simulink model "Exp5_AtoD_Soham_19EE10075"  (R2020b)
settings: Solver=VariableStepAuto  StartTime=0.0  StopTime=10.0  RelTol=1e-3
libraries: powerlib x40, powerlib_meascontrol x10
settings Model: Creator=User  LastModifiedBy=User

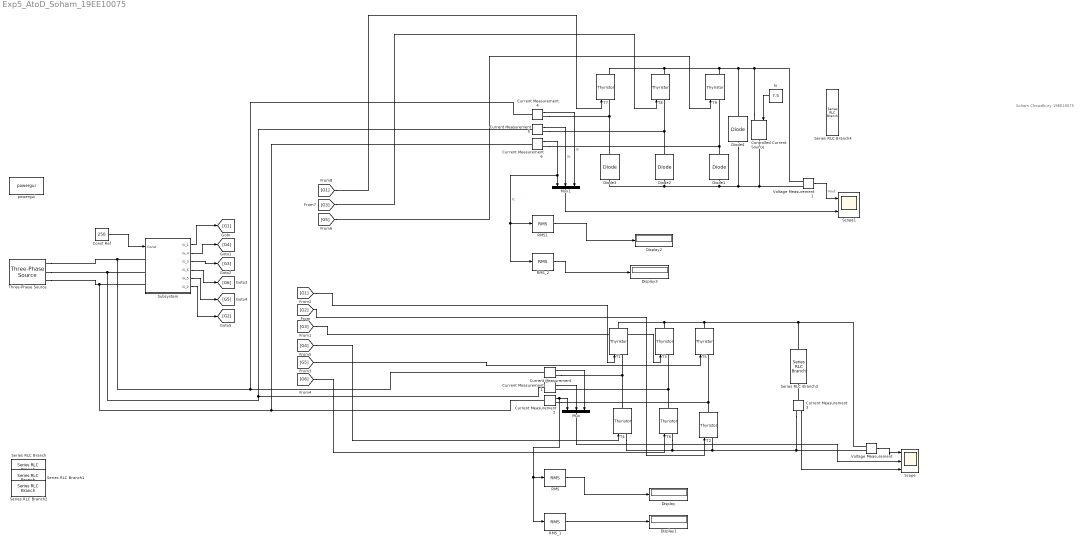
== system Exp5_AtoD_Soham_19EE10075 ==
  note: Soham Chowdhury
      | 19EE10075
  Const Ref : Constant  Value=250
  Controlled Current Source : powerlib/Electrical Sources/Controlled Current Source  Initialize=on  Source_Type=DC  Amplitude=7.5  Phase=0  Frequency=0  Measurements=None
  Current Measurement{,1..6} (7 alike) : powerlib/Measurements/Current Measurement  PhasorSimulation=off  OutputType=Complex  PSBequivalent=0
  Diode{1..4} (4 alike) : powerlib/Power Electronics/Diode  Ron=1e-3  Lon=0  Vf=0  IC=0  UseSnubber=0  Rs=1e12  Cs=inf  Measurements=off
  Display{,1..3} (4 alike) : Display
  Io : Constant  Value=7.5
  Mux : Mux  Inputs=3
  Mux1 : Mux  Inputs=3
  RMS : powerlib_meascontrol/Measurements/RMS  TrueRMS=on  Freq=50  RMSInit=0  Ts=0
  RMS1 : powerlib_meascontrol/Measurements/RMS  TrueRMS=on  Freq=50  RMSInit=0  Ts=0
  RMS_1 : powerlib_meascontrol/Measurements/RMS  TrueRMS=off  Freq=50  RMSInit=0  Ts=0
  RMS_2 : powerlib_meascontrol/Measurements/RMS  TrueRMS=off  Freq=50  RMSInit=0  Ts=0
  Scope : Scope  NumInputPorts=3
  Scope1 : Scope  NumInputPorts=2
  Series RLC Branch : powerlib/Elements/Series RLC Branch  LConnTagsString=__new0  RConnTagsString=__new0  BranchType=L  Resistance=1  Inductance=5e-3  SetiL0=off  InitialCurrent=0  Capacitance=1e-6  Setx0=off  InitialVoltage=0  Measurements=None
  Series RLC Branch1 : powerlib/Elements/Series RLC Branch  LConnTagsString=__new0  RConnTagsString=__new0  BranchType=L  Resistance=1  Inductance=5e-3  SetiL0=off  InitialCurrent=0  Capacitance=1e-6  Setx0=off  InitialVoltage=0  Measurements=None
  Series RLC Branch2 : powerlib/Elements/Series RLC Branch  LConnTagsString=__new0  RConnTagsString=__new0  BranchType=L  Resistance=1  Inductance=5e-3  SetiL0=off  InitialCurrent=0  Capacitance=1e-6  Setx0=off  InitialVoltage=0  Measurements=None
  Series RLC Branch3 : powerlib/Elements/Series RLC Branch  LConnTagsString=__new0  RConnTagsString=__new0  BranchType=RL  Resistance=1  Inductance=60e-3  SetiL0=off  InitialCurrent=0  Capacitance=1e-6  Setx0=off  InitialVoltage=0  Measurements=None
  Series RLC Branch4 : powerlib/Elements/Series RLC Branch  LConnTagsString=__new0  RConnTagsString=__new0  BranchType=RL  Resistance=29.18  Inductance=50e-3  SetiL0=off  InitialCurrent=0  Capacitance=1e-6  Setx0=off  InitialVoltage=0  Measurements=None
  Subsystem : Subsystem
  T{1..6} (6 alike) : powerlib/Power Electronics/Thyristor  Ron=1e-3  Lon=0  Vf=0  IC=0  Rs=1e12  Cs=inf  Measurements=off
  T7 : powerlib/Power Electronics/Thyristor  Ron=1e-3  Lon=0  Vf=0  IC=0  Rs=1e12  Cs=inf  Measurements=on
  T8 : powerlib/Power Electronics/Thyristor  Ron=1e-3  Lon=0  Vf=0  IC=0  Rs=1e12  Cs=inf  Measurements=on
  T9 : powerlib/Power Electronics/Thyristor  Ron=1e-3  Lon=0  Vf=0  IC=0  Rs=1e12  Cs=inf  Measurements=on
  Three-Phase Source : powerlib/Electrical Sources/Three-Phase Source  InternalConnection=Y  VoltagePhases=off  Voltage=220  PhaseAngle=0  Voltage_phases=[25e3 25e3 25e3]/sqrt(3)  PhaseAngles_phases=[0 -120 +120]  Frequency=50  NonIdealSource=on  SpecifyImpedance=off  Resistance=0  Inductance=0  ShortCircuitLevel=100e6  BaseVoltage=220  XRratio=7  BusType=swing  Pref=10e3  Qref=0  Prefabc=[10e3, 10e3, 10e3]  Qrefabc=[0, 0, 0]  Qmin=-inf  Qmax=inf
  Voltage Measurement : powerlib/Measurements/Voltage Measurement  PhasorSimulation=off  OutputType=Complex  PSBequivalent=0
  Voltage Measurement1 : powerlib/Measurements/Voltage Measurement  PhasorSimulation=off  OutputType=Complex  PSBequivalent=0
  powergui : powerlib/powergui  Priority=1  SimulationMode=Continuous  SampleTime=1e-9  frequency=60  Iterations=50  frequencyindice=50  Pbase=100e6  ErrMax=1e-4  UnitsV=kV  UnitsW=MW  buscounter=0  FunctionMessages=off  echomessages=off  EnableUseOfTLC=off  CurrentSourceSwitches=off  DisableSnubberDevices=off  DisableRonSwitches=off  DisableVfSwitches=off  DisplayEquations=off  AutomaticDiscreteSolvers=off  SolverType=Tustin/Backward Euler (TBE)  Interpol=off  ExternalGateDelay=off  methode=off  Ts=100  x0status=blocks  SPID=on  SwTol=0  HookPort=off  NonlinearTolerance=1e-4  nMaxIteration=100  ContinueOnMaxIteration=off  RestoreLinks=warning  ResistiveCurrentMeasurement=off  Frange=[0:2:500]  Ylog=off  Xlog=on  ShowGrid=off  save=off  variable=ZData  structure=0  ZoomFFT=off  StartTime=0.0  cycles=1  DisplayStyle=1  fundamental=60  FreqAxis=off  MaxFrequency=1000  frequencyindicesteady=1  RmsSteady=1  display=off
  wires:
  [G1] -> T7/1
  RMS_2/1 -> Display3/1
  Voltage Measurement1/1 -> Scope1/1  "Vout"
  Current Measurement4/1 -> Mux1/3  "Ia"
  Mux1/1 -> Scope1/2
  Current Measurement6/1 -> RMS1/1, RMS_2/1, Mux1/1  "Ic"
  Io/1 -> Controlled Current Source/1
  [G5] -> T9/1
  [G2] -> T2/1
  [G1] -> T1/1
  Mux/1 -> Scope/2
  Current Measurement1/1 -> Mux/2
  Current Measurement3/1 -> Scope/3
  Current Measurement5/1 -> Mux1/2  "Ib"
  RMS_1/1 -> Display1/1
  RMS/1 -> Display/1
  [G5] -> T5/1
  [G4] -> T4/1
  Current Measurement/1 -> Mux/3
  RMS1/1 -> Display2/1
  Current Measurement2/1 -> Mux/1, RMS_1/1, RMS/1
  Subsystem/6(G_2) -> [G2]
  Subsystem/2(G_4) -> [G4]
  Subsystem/5(G_5) -> [G5]
  Subsystem/1(G_1) -> [G1]
  Const Ref/1 -> Subsystem/1(Const)
  Voltage Measurement/1 -> Scope/1
  Subsystem/3(G_3) -> [G3]
  Subsystem/4(G_6) -> [G6]
  [G6] -> T6/1
  [G3] -> T8/1
  [G3] -> T3/1
  connections:
  Controlled Current Source/LConn1 -- Voltage Measurement1/LConn1 -- Diode4/RConn1 -- T7/RConn1 -- T8/RConn1 -- T9/RConn1
  Diode1/LConn1 -- Voltage Measurement1/LConn2 -- Controlled Current Source/RConn1 -- Diode4/LConn1 -- Diode2/LConn1 -- Diode3/LConn1
  Current Measurement6/RConn1 -- Diode1/RConn1 -- T9/LConn1
  T1/RConn1 -- T3/RConn1 -- T5/RConn1 -- Series RLC Branch3/LConn1 -- Voltage Measurement/LConn1
  T1/LConn1 -- T4/RConn1 -- Current Measurement/RConn1
  Current Measurement1/LConn1 -- Current Measurement5/LConn1 -- Subsystem/LConn2 -- Three-Phase Source/RConn2
  T2/LConn1 -- Voltage Measurement/LConn2 -- Current Measurement3/RConn1 -- T4/LConn1 -- T6/LConn1
  Three-Phase Source/RConn1 -- Current Measurement4/LConn1 -- Current Measurement/LConn1 -- Subsystem/LConn1
  T5/LConn1 -- T2/RConn1 -- Current Measurement2/RConn1
  Three-Phase Source/RConn3 -- Current Measurement6/LConn1 -- Current Measurement2/LConn1 -- Subsystem/LConn3
  Current Measurement5/RConn1 -- T8/LConn1 -- Diode2/RConn1
  Current Measurement4/RConn1 -- T7/LConn1 -- Diode3/RConn1
  T3/LConn1 -- T6/RConn1 -- Current Measurement1/RConn1
  Current Measurement3/LConn1 -- Series RLC Branch3/RConn1

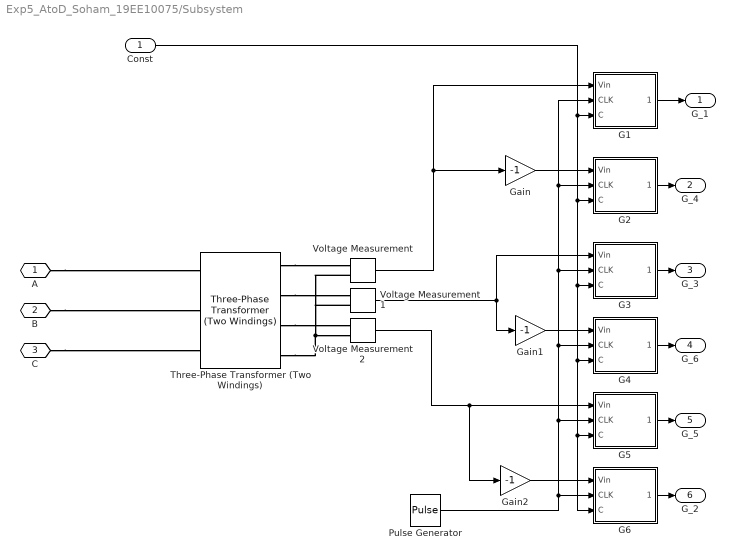
== system Exp5_AtoD_Soham_19EE10075/Subsystem ==
  Const : Inport
  G1 : Subsystem
  G2 : Subsystem
  G3 : Subsystem
  G4 : Subsystem
  G5 : Subsystem
  G6 : Subsystem
  Gain : Gain  Gain=-1
  Gain1 : Gain  Gain=-1
  Gain2 : Gain  Gain=-1
  Pulse Generator : DiscretePulseGenerator  PulseType=Time based  Period=1e-5  PulseWidth=50
  Three-Phase Transformer (Two Windings) : powerlib/Elements/Three-Phase Transformer (Two Windings)  Winding1Connection=Y  Winding2Connection=Yn  CoreType=Three single-phase transformers  SetSaturation=off  Hysteresis=off  DataFile='hysteresis'  SetInitialFlux=off  Measurements=None  UNITS=SI  NominalPower=[100 , 50 ]  Winding1=[220*sqrt(2) 0 0]  Winding2=[5*sqrt(3) 0 0]  Rm=1e6  Lm=1e6  L0=2.866  Saturation=[0 0;0.66653 1910.3;277.72 2419.7]  InitialFluxes=[1273.5 -1273.5 1114.3]  BreakLoop=off  DiscreteSolver=Trapezoidal iterative  DataType=on  TransfoNumber=1
  Voltage Measurement : powerlib/Measurements/Voltage Measurement  PhasorSimulation=off  OutputType=Complex  PSBequivalent=0
  Voltage Measurement1 : powerlib/Measurements/Voltage Measurement  PhasorSimulation=off  OutputType=Complex  PSBequivalent=0
  Voltage Measurement2 : powerlib/Measurements/Voltage Measurement  PhasorSimulation=off  OutputType=Complex  PSBequivalent=0
  A : PMIOPort  Side=Left
  B : PMIOPort  Port=2  Side=Left
  C : PMIOPort  Port=3  Side=Left
  G_1 : Outport
  G_4 : Outport  Port=2
  G_3 : Outport  Port=3
  G_6 : Outport  Port=4
  G_5 : Outport  Port=5
  G_2 : Outport  Port=6
  wires:
  Voltage Measurement/1 -> Gain/1, G1/1(Vin)
  Voltage Measurement2/1 -> G5/1(Vin), Gain2/1
  Const/1 -> G2/3(C), G3/3(C), G4/3(C), G6/3(C), G5/3(C), G1/3(C)
  G2/1(Outport) -> G_4/1
  Pulse Generator/1 -> G6/2(CLK), G5/2(CLK), G4/2(CLK), G3/2(CLK), G2/2(CLK), G1/2(CLK)
  G4/1(Outport) -> G_6/1
  Voltage Measurement1/1 -> G3/1(Vin), Gain1/1
  G6/1(Outport) -> G_2/1
  Gain2/1 -> G6/1(Vin)
  Gain/1 -> G2/1(Vin)
  Gain1/1 -> G4/1(Vin)
  G3/1(Outport) -> G_3/1
  G5/1(Outport) -> G_5/1
  G1/1(Outport) -> G_1/1
  connections:
  Three-Phase Transformer (Two Windings)/RConn1 -- Voltage Measurement/LConn1
  Three-Phase Transformer (Two Windings)/RConn4 -- Voltage Measurement/LConn2 -- Voltage Measurement1/LConn2 -- Voltage Measurement2/LConn2
  Three-Phase Transformer (Two Windings)/RConn2 -- Voltage Measurement1/LConn1
  B/RConn1 -- Three-Phase Transformer (Two Windings)/LConn2
  Three-Phase Transformer (Two Windings)/RConn3 -- Voltage Measurement2/LConn1
  C/RConn1 -- Three-Phase Transformer (Two Windings)/LConn3
  A/RConn1 -- Three-Phase Transformer (Two Windings)/LConn1

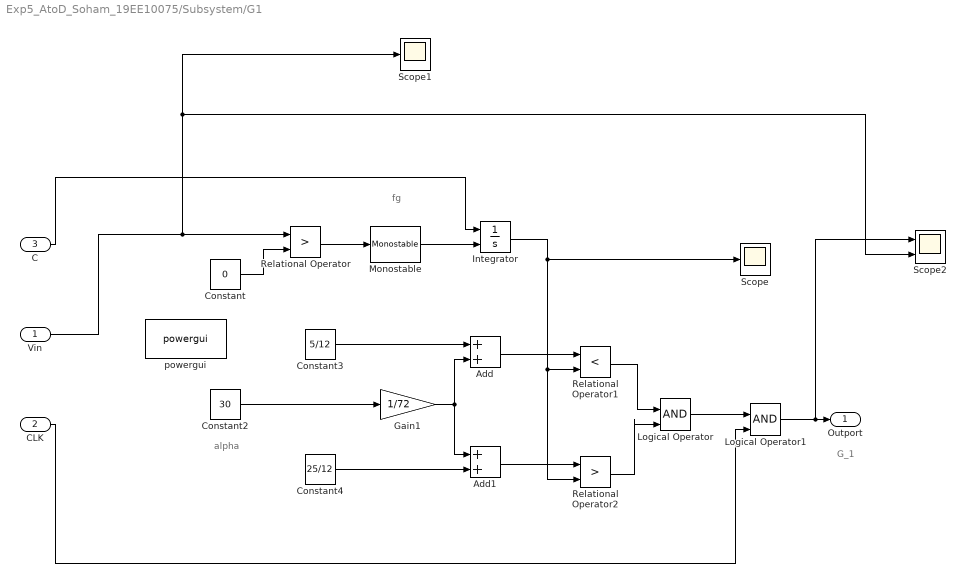
== system Exp5_AtoD_Soham_19EE10075/Subsystem/G1 ==
  note: G_1
  note: alpha
  note: fg
  Vin : Inport
  CLK : Inport  Port=2
  C : Inport  Port=3
  Add : Sum
  Add1 : Sum
  Constant : Constant  Value=0
  Constant2 : Constant  Value=30
  Constant3 : Constant  Value=5/12
  Constant4 : Constant  Value=25/12
  Gain1 : Gain  Gain=1/72
  Integrator : Integrator  ExternalReset=rising
  Logical Operator : Logic  IconShape=distinctive  AllPortsSameDT=off  OutDataTypeStr=boolean
  Logical Operator1 : Logic  IconShape=distinctive  AllPortsSameDT=off  OutDataTypeStr=boolean
  Monostable : powerlib_meascontrol/Logic/Monostable  EdgeDetect=Rising  PulseDuration=1e-05  ic=0  Ts=0
      settings: SourceProductBaseCode=PS
  Relational Operator : RelationalOperator  Operator=>  OutDataTypeStr=boolean  RndMeth=Simplest
  Relational Operator1 : RelationalOperator  Operator=<  OutDataTypeStr=boolean  RndMeth=Simplest
  Relational Operator2 : RelationalOperator  Operator=>  OutDataTypeStr=boolean  RndMeth=Simplest
  Scope : Scope
  Scope1 : Scope
  Scope2 : Scope  NumInputPorts=2
  powergui : powerlib/powergui  Priority=1  SimulationMode=Discrete  SampleTime=1e-9  frequency=60  Iterations=50  frequencyindice=60  Pbase=100e6  ErrMax=1e-4  UnitsV=kV  UnitsW=MW  buscounter=0  FunctionMessages=off  echomessages=off  EnableUseOfTLC=off  CurrentSourceSwitches=off  DisableSnubberDevices=off  DisableRonSwitches=off  DisableVfSwitches=off  DisplayEquations=off  AutomaticDiscreteSolvers=off  SolverType=Tustin/Backward Euler (TBE)  Interpol=off  ExternalGateDelay=off  methode=off  Ts=100  x0status=blocks  SPID=on  SwTol=0  HookPort=off  NonlinearTolerance=1e-4  nMaxIteration=100  ContinueOnMaxIteration=off  RestoreLinks=warning  ResistiveCurrentMeasurement=off  Frange=[0:2:500]  Ylog=off  Xlog=on  ShowGrid=off  save=off  variable=ZData  structure=0  ZoomFFT=off  StartTime=0.0  cycles=1  DisplayStyle=1  fundamental=60  FreqAxis=off  MaxFrequency=1000  frequencyindicesteady=1  RmsSteady=1  display=off
  Outport : Outport
  wires:
  Add1/1 -> Relational Operator2/1
  Integrator/1 -> Relational Operator2/2, Relational Operator1/2, Scope/1
  Relational Operator/1 -> Monostable/1
  Add/1 -> Relational Operator1/1
  Constant/1 -> Relational Operator/2
  Relational Operator2/1 -> Logical Operator/2
  Constant3/1 -> Add/1
  Gain1/1 -> Add1/1, Add/2
  Constant4/1 -> Add1/2
  Logical Operator/1 -> Logical Operator1/1
  Monostable/1 -> Integrator/2
  Relational Operator1/1 -> Logical Operator/1
  Logical Operator1/1 -> Scope2/1, Outport/1
  Vin/1 -> Scope2/2, Scope1/1, Relational Operator/1
  CLK/1 -> Logical Operator1/2
  C/1 -> Integrator/1
  Constant2/1 -> Gain1/1

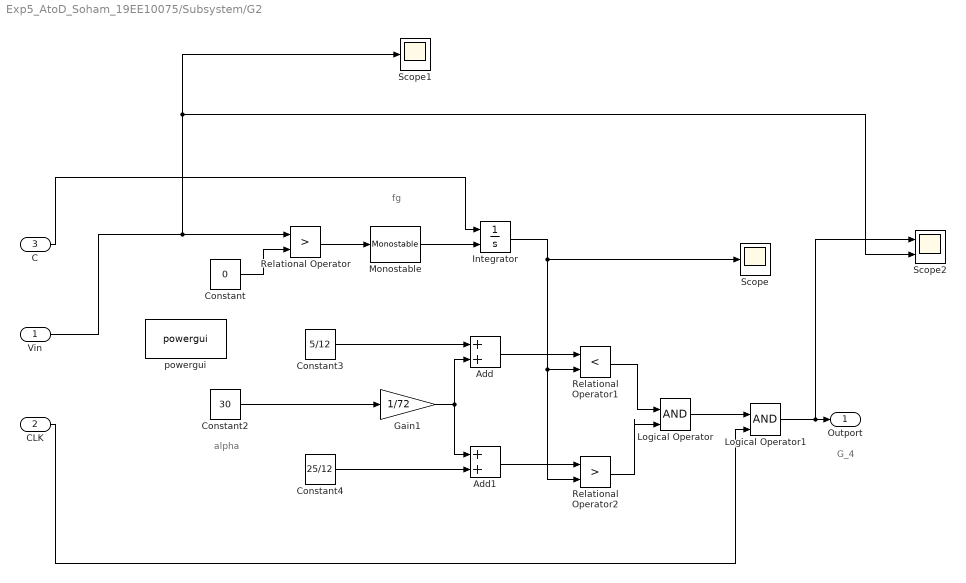
== system Exp5_AtoD_Soham_19EE10075/Subsystem/G2 ==
  note: G_4
  note: alpha
  note: fg
  Vin : Inport
  CLK : Inport  Port=2
  C : Inport  Port=3
  Add : Sum
  Add1 : Sum
  Constant : Constant  Value=0
  Constant2 : Constant  Value=30
  Constant3 : Constant  Value=5/12
  Constant4 : Constant  Value=25/12
  Gain1 : Gain  Gain=1/72
  Integrator : Integrator  ExternalReset=rising
  Logical Operator : Logic  IconShape=distinctive  AllPortsSameDT=off  OutDataTypeStr=boolean
  Logical Operator1 : Logic  IconShape=distinctive  AllPortsSameDT=off  OutDataTypeStr=boolean
  Monostable : powerlib_meascontrol/Logic/Monostable  EdgeDetect=Rising  PulseDuration=1e-05  ic=0  Ts=0
      settings: SourceProductBaseCode=PS
  Relational Operator : RelationalOperator  Operator=>  OutDataTypeStr=boolean  RndMeth=Simplest
  Relational Operator1 : RelationalOperator  Operator=<  OutDataTypeStr=boolean  RndMeth=Simplest
  Relational Operator2 : RelationalOperator  Operator=>  OutDataTypeStr=boolean  RndMeth=Simplest
  Scope : Scope
  Scope1 : Scope
  Scope2 : Scope  NumInputPorts=2
  powergui : powerlib/powergui  Priority=1  SimulationMode=Discrete  SampleTime=1e-9  frequency=60  Iterations=50  frequencyindice=60  Pbase=100e6  ErrMax=1e-4  UnitsV=kV  UnitsW=MW  buscounter=0  FunctionMessages=off  echomessages=off  EnableUseOfTLC=off  CurrentSourceSwitches=off  DisableSnubberDevices=off  DisableRonSwitches=off  DisableVfSwitches=off  DisplayEquations=off  AutomaticDiscreteSolvers=off  SolverType=Tustin/Backward Euler (TBE)  Interpol=off  ExternalGateDelay=off  methode=off  Ts=100  x0status=blocks  SPID=on  SwTol=0  HookPort=off  NonlinearTolerance=1e-4  nMaxIteration=100  ContinueOnMaxIteration=off  RestoreLinks=warning  ResistiveCurrentMeasurement=off  Frange=[0:2:500]  Ylog=off  Xlog=on  ShowGrid=off  save=off  variable=ZData  structure=0  ZoomFFT=off  StartTime=0.0  cycles=1  DisplayStyle=1  fundamental=60  FreqAxis=off  MaxFrequency=1000  frequencyindicesteady=1  RmsSteady=1  display=off
  Outport : Outport
  wires:
  Add1/1 -> Relational Operator2/1
  Integrator/1 -> Relational Operator2/2, Relational Operator1/2, Scope/1
  Relational Operator/1 -> Monostable/1
  Add/1 -> Relational Operator1/1
  Constant/1 -> Relational Operator/2
  Relational Operator2/1 -> Logical Operator/2
  Constant3/1 -> Add/1
  Gain1/1 -> Add1/1, Add/2
  Constant4/1 -> Add1/2
  Logical Operator/1 -> Logical Operator1/1
  Monostable/1 -> Integrator/2
  Relational Operator1/1 -> Logical Operator/1
  Logical Operator1/1 -> Scope2/1, Outport/1
  Vin/1 -> Scope2/2, Scope1/1, Relational Operator/1
  CLK/1 -> Logical Operator1/2
  C/1 -> Integrator/1
  Constant2/1 -> Gain1/1

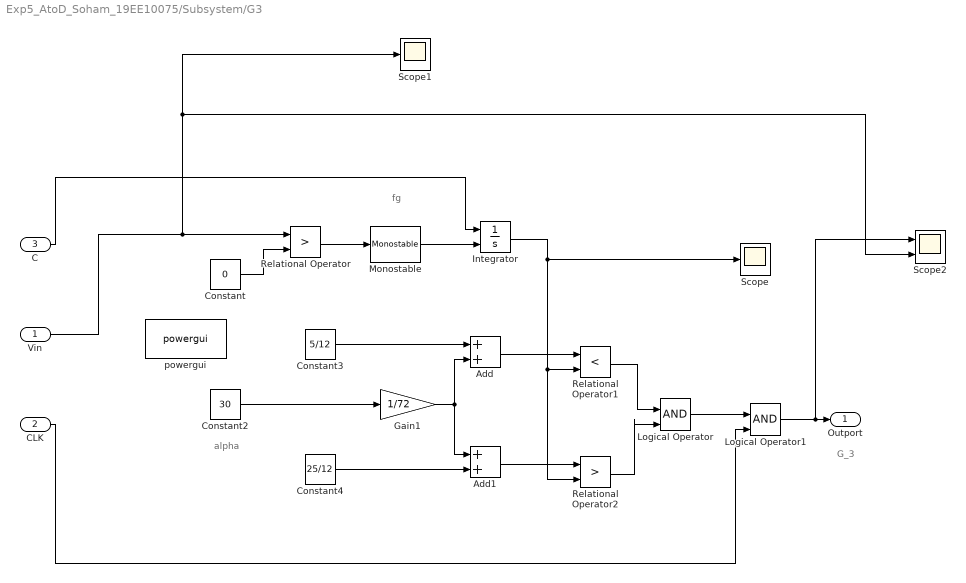
== system Exp5_AtoD_Soham_19EE10075/Subsystem/G3 ==
  note: G_3
  note: alpha
  note: fg
  Vin : Inport
  CLK : Inport  Port=2
  C : Inport  Port=3
  Add : Sum
  Add1 : Sum
  Constant : Constant  Value=0
  Constant2 : Constant  Value=30
  Constant3 : Constant  Value=5/12
  Constant4 : Constant  Value=25/12
  Gain1 : Gain  Gain=1/72
  Integrator : Integrator  ExternalReset=rising
  Logical Operator : Logic  IconShape=distinctive  AllPortsSameDT=off  OutDataTypeStr=boolean
  Logical Operator1 : Logic  IconShape=distinctive  AllPortsSameDT=off  OutDataTypeStr=boolean
  Monostable : powerlib_meascontrol/Logic/Monostable  EdgeDetect=Rising  PulseDuration=1e-05  ic=0  Ts=0
      settings: SourceProductBaseCode=PS
  Relational Operator : RelationalOperator  Operator=>  OutDataTypeStr=boolean  RndMeth=Simplest
  Relational Operator1 : RelationalOperator  Operator=<  OutDataTypeStr=boolean  RndMeth=Simplest
  Relational Operator2 : RelationalOperator  Operator=>  OutDataTypeStr=boolean  RndMeth=Simplest
  Scope : Scope
  Scope1 : Scope
  Scope2 : Scope  NumInputPorts=2
  powergui : powerlib/powergui  Priority=1  SimulationMode=Discrete  SampleTime=1e-9  frequency=60  Iterations=50  frequencyindice=60  Pbase=100e6  ErrMax=1e-4  UnitsV=kV  UnitsW=MW  buscounter=0  FunctionMessages=off  echomessages=off  EnableUseOfTLC=off  CurrentSourceSwitches=off  DisableSnubberDevices=off  DisableRonSwitches=off  DisableVfSwitches=off  DisplayEquations=off  AutomaticDiscreteSolvers=off  SolverType=Tustin/Backward Euler (TBE)  Interpol=off  ExternalGateDelay=off  methode=off  Ts=100  x0status=blocks  SPID=on  SwTol=0  HookPort=off  NonlinearTolerance=1e-4  nMaxIteration=100  ContinueOnMaxIteration=off  RestoreLinks=warning  ResistiveCurrentMeasurement=off  Frange=[0:2:500]  Ylog=off  Xlog=on  ShowGrid=off  save=off  variable=ZData  structure=0  ZoomFFT=off  StartTime=0.0  cycles=1  DisplayStyle=1  fundamental=60  FreqAxis=off  MaxFrequency=1000  frequencyindicesteady=1  RmsSteady=1  display=off
  Outport : Outport
  wires:
  Add1/1 -> Relational Operator2/1
  Integrator/1 -> Relational Operator2/2, Relational Operator1/2, Scope/1
  Relational Operator/1 -> Monostable/1
  Add/1 -> Relational Operator1/1
  Constant/1 -> Relational Operator/2
  Relational Operator2/1 -> Logical Operator/2
  Constant3/1 -> Add/1
  Gain1/1 -> Add1/1, Add/2
  Constant4/1 -> Add1/2
  Logical Operator/1 -> Logical Operator1/1
  Monostable/1 -> Integrator/2
  Relational Operator1/1 -> Logical Operator/1
  Logical Operator1/1 -> Scope2/1, Outport/1
  Vin/1 -> Scope2/2, Scope1/1, Relational Operator/1
  CLK/1 -> Logical Operator1/2
  C/1 -> Integrator/1
  Constant2/1 -> Gain1/1

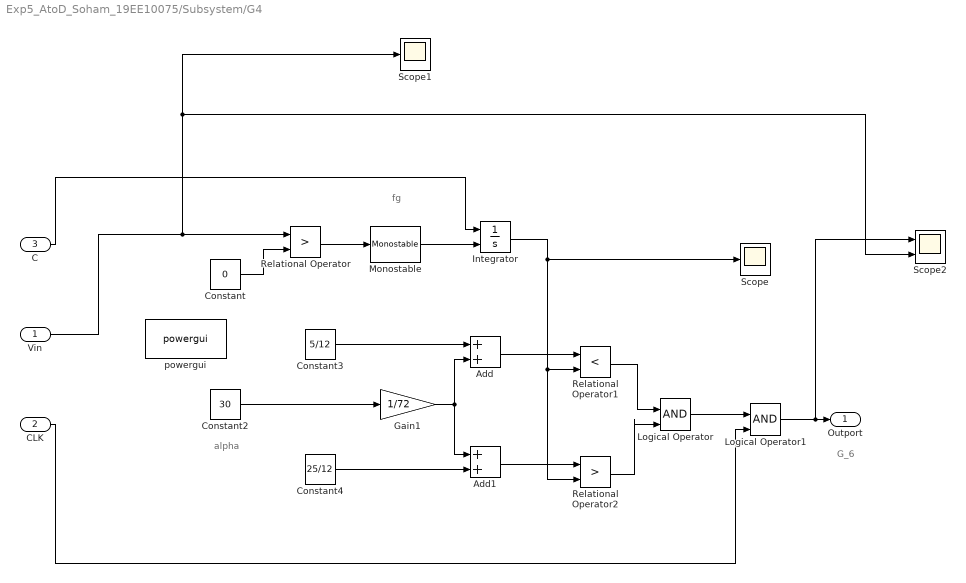
== system Exp5_AtoD_Soham_19EE10075/Subsystem/G4 ==
  note: G_6
  note: alpha
  note: fg
  Vin : Inport
  CLK : Inport  Port=2
  C : Inport  Port=3
  Add : Sum
  Add1 : Sum
  Constant : Constant  Value=0
  Constant2 : Constant  Value=30
  Constant3 : Constant  Value=5/12
  Constant4 : Constant  Value=25/12
  Gain1 : Gain  Gain=1/72
  Integrator : Integrator  ExternalReset=rising
  Logical Operator : Logic  IconShape=distinctive  AllPortsSameDT=off  OutDataTypeStr=boolean
  Logical Operator1 : Logic  IconShape=distinctive  AllPortsSameDT=off  OutDataTypeStr=boolean
  Monostable : powerlib_meascontrol/Logic/Monostable  EdgeDetect=Rising  PulseDuration=1e-05  ic=0  Ts=0
      settings: SourceProductBaseCode=PS
  Relational Operator : RelationalOperator  Operator=>  OutDataTypeStr=boolean  RndMeth=Simplest
  Relational Operator1 : RelationalOperator  Operator=<  OutDataTypeStr=boolean  RndMeth=Simplest
  Relational Operator2 : RelationalOperator  Operator=>  OutDataTypeStr=boolean  RndMeth=Simplest
  Scope : Scope
  Scope1 : Scope
  Scope2 : Scope  NumInputPorts=2
  powergui : powerlib/powergui  Priority=1  SimulationMode=Discrete  SampleTime=1e-9  frequency=60  Iterations=50  frequencyindice=60  Pbase=100e6  ErrMax=1e-4  UnitsV=kV  UnitsW=MW  buscounter=0  FunctionMessages=off  echomessages=off  EnableUseOfTLC=off  CurrentSourceSwitches=off  DisableSnubberDevices=off  DisableRonSwitches=off  DisableVfSwitches=off  DisplayEquations=off  AutomaticDiscreteSolvers=off  SolverType=Tustin/Backward Euler (TBE)  Interpol=off  ExternalGateDelay=off  methode=off  Ts=100  x0status=blocks  SPID=on  SwTol=0  HookPort=off  NonlinearTolerance=1e-4  nMaxIteration=100  ContinueOnMaxIteration=off  RestoreLinks=warning  ResistiveCurrentMeasurement=off  Frange=[0:2:500]  Ylog=off  Xlog=on  ShowGrid=off  save=off  variable=ZData  structure=0  ZoomFFT=off  StartTime=0.0  cycles=1  DisplayStyle=1  fundamental=60  FreqAxis=off  MaxFrequency=1000  frequencyindicesteady=1  RmsSteady=1  display=off
  Outport : Outport
  wires:
  Add1/1 -> Relational Operator2/1
  Integrator/1 -> Relational Operator2/2, Relational Operator1/2, Scope/1
  Relational Operator/1 -> Monostable/1
  Add/1 -> Relational Operator1/1
  Constant/1 -> Relational Operator/2
  Relational Operator2/1 -> Logical Operator/2
  Constant3/1 -> Add/1
  Gain1/1 -> Add1/1, Add/2
  Constant4/1 -> Add1/2
  Logical Operator/1 -> Logical Operator1/1
  Monostable/1 -> Integrator/2
  Relational Operator1/1 -> Logical Operator/1
  Logical Operator1/1 -> Scope2/1, Outport/1
  Vin/1 -> Scope2/2, Scope1/1, Relational Operator/1
  CLK/1 -> Logical Operator1/2
  C/1 -> Integrator/1
  Constant2/1 -> Gain1/1

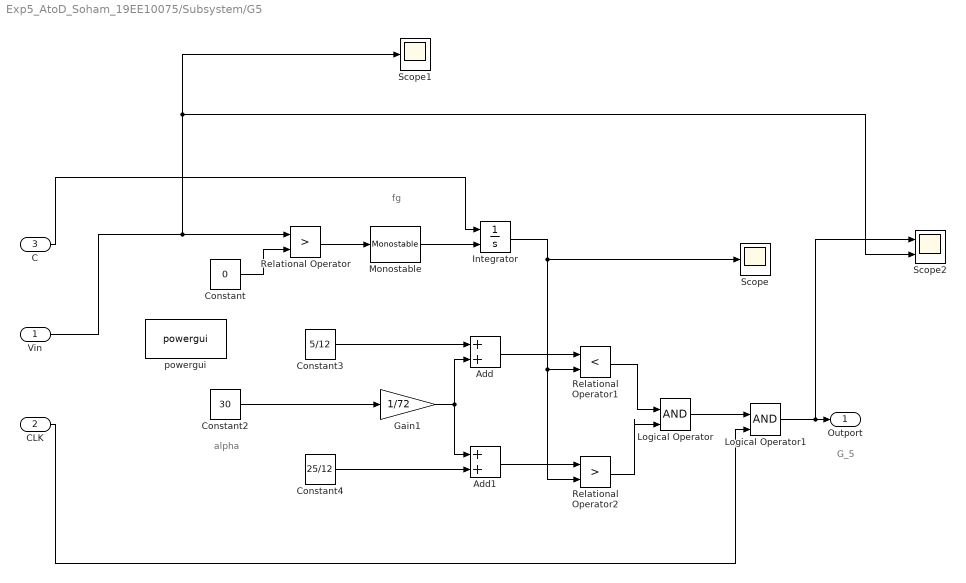
== system Exp5_AtoD_Soham_19EE10075/Subsystem/G5 ==
  note: G_5
  note: alpha
  note: fg
  Vin : Inport
  CLK : Inport  Port=2
  C : Inport  Port=3
  Add : Sum
  Add1 : Sum
  Constant : Constant  Value=0
  Constant2 : Constant  Value=30
  Constant3 : Constant  Value=5/12
  Constant4 : Constant  Value=25/12
  Gain1 : Gain  Gain=1/72
  Integrator : Integrator  ExternalReset=rising
  Logical Operator : Logic  IconShape=distinctive  AllPortsSameDT=off  OutDataTypeStr=boolean
  Logical Operator1 : Logic  IconShape=distinctive  AllPortsSameDT=off  OutDataTypeStr=boolean
  Monostable : powerlib_meascontrol/Logic/Monostable  EdgeDetect=Rising  PulseDuration=1e-05  ic=0  Ts=0
      settings: SourceProductBaseCode=PS
  Relational Operator : RelationalOperator  Operator=>  OutDataTypeStr=boolean  RndMeth=Simplest
  Relational Operator1 : RelationalOperator  Operator=<  OutDataTypeStr=boolean  RndMeth=Simplest
  Relational Operator2 : RelationalOperator  Operator=>  OutDataTypeStr=boolean  RndMeth=Simplest
  Scope : Scope
  Scope1 : Scope
  Scope2 : Scope  NumInputPorts=2
  powergui : powerlib/powergui  Priority=1  SimulationMode=Discrete  SampleTime=1e-9  frequency=60  Iterations=50  frequencyindice=60  Pbase=100e6  ErrMax=1e-4  UnitsV=kV  UnitsW=MW  buscounter=0  FunctionMessages=off  echomessages=off  EnableUseOfTLC=off  CurrentSourceSwitches=off  DisableSnubberDevices=off  DisableRonSwitches=off  DisableVfSwitches=off  DisplayEquations=off  AutomaticDiscreteSolvers=off  SolverType=Tustin/Backward Euler (TBE)  Interpol=off  ExternalGateDelay=off  methode=off  Ts=100  x0status=blocks  SPID=on  SwTol=0  HookPort=off  NonlinearTolerance=1e-4  nMaxIteration=100  ContinueOnMaxIteration=off  RestoreLinks=warning  ResistiveCurrentMeasurement=off  Frange=[0:2:500]  Ylog=off  Xlog=on  ShowGrid=off  save=off  variable=ZData  structure=0  ZoomFFT=off  StartTime=0.0  cycles=1  DisplayStyle=1  fundamental=60  FreqAxis=off  MaxFrequency=1000  frequencyindicesteady=1  RmsSteady=1  display=off
  Outport : Outport
  wires:
  Add1/1 -> Relational Operator2/1
  Integrator/1 -> Relational Operator2/2, Relational Operator1/2, Scope/1
  Relational Operator/1 -> Monostable/1
  Add/1 -> Relational Operator1/1
  Constant/1 -> Relational Operator/2
  Relational Operator2/1 -> Logical Operator/2
  Constant3/1 -> Add/1
  Gain1/1 -> Add1/1, Add/2
  Constant4/1 -> Add1/2
  Logical Operator/1 -> Logical Operator1/1
  Monostable/1 -> Integrator/2
  Relational Operator1/1 -> Logical Operator/1
  Logical Operator1/1 -> Scope2/1, Outport/1
  Vin/1 -> Scope2/2, Scope1/1, Relational Operator/1
  CLK/1 -> Logical Operator1/2
  C/1 -> Integrator/1
  Constant2/1 -> Gain1/1

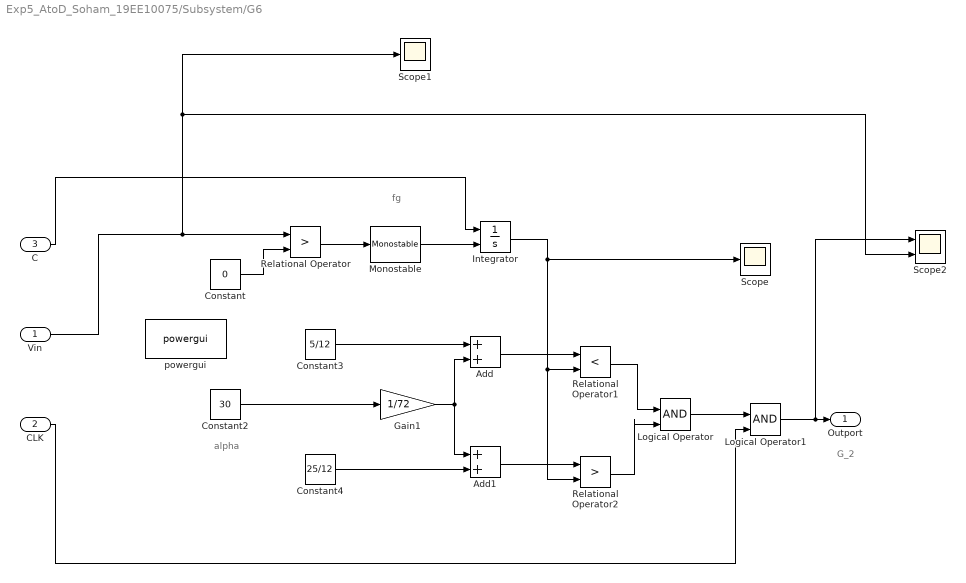
== system Exp5_AtoD_Soham_19EE10075/Subsystem/G6 ==
  note: G_2
  note: alpha
  note: fg
  Vin : Inport
  CLK : Inport  Port=2
  C : Inport  Port=3
  Add : Sum
  Add1 : Sum
  Constant : Constant  Value=0
  Constant2 : Constant  Value=30
  Constant3 : Constant  Value=5/12
  Constant4 : Constant  Value=25/12
  Gain1 : Gain  Gain=1/72
  Integrator : Integrator  ExternalReset=rising
  Logical Operator : Logic  IconShape=distinctive  AllPortsSameDT=off  OutDataTypeStr=boolean
  Logical Operator1 : Logic  IconShape=distinctive  AllPortsSameDT=off  OutDataTypeStr=boolean
  Monostable : powerlib_meascontrol/Logic/Monostable  EdgeDetect=Rising  PulseDuration=1e-05  ic=0  Ts=0
      settings: SourceProductBaseCode=PS
  Relational Operator : RelationalOperator  Operator=>  OutDataTypeStr=boolean  RndMeth=Simplest
  Relational Operator1 : RelationalOperator  Operator=<  OutDataTypeStr=boolean  RndMeth=Simplest
  Relational Operator2 : RelationalOperator  Operator=>  OutDataTypeStr=boolean  RndMeth=Simplest
  Scope : Scope
  Scope1 : Scope
  Scope2 : Scope  NumInputPorts=2
  powergui : powerlib/powergui  Priority=1  SimulationMode=Discrete  SampleTime=1e-9  frequency=60  Iterations=50  frequencyindice=60  Pbase=100e6  ErrMax=1e-4  UnitsV=kV  UnitsW=MW  buscounter=0  FunctionMessages=off  echomessages=off  EnableUseOfTLC=off  CurrentSourceSwitches=off  DisableSnubberDevices=off  DisableRonSwitches=off  DisableVfSwitches=off  DisplayEquations=off  AutomaticDiscreteSolvers=off  SolverType=Tustin/Backward Euler (TBE)  Interpol=off  ExternalGateDelay=off  methode=off  Ts=100  x0status=blocks  SPID=on  SwTol=0  HookPort=off  NonlinearTolerance=1e-4  nMaxIteration=100  ContinueOnMaxIteration=off  RestoreLinks=warning  ResistiveCurrentMeasurement=off  Frange=[0:2:500]  Ylog=off  Xlog=on  ShowGrid=off  save=off  variable=ZData  structure=0  ZoomFFT=off  StartTime=0.0  cycles=1  DisplayStyle=1  fundamental=60  FreqAxis=off  MaxFrequency=1000  frequencyindicesteady=1  RmsSteady=1  display=off
  Outport : Outport
  wires:
  Add1/1 -> Relational Operator2/1
  Integrator/1 -> Relational Operator2/2, Relational Operator1/2, Scope/1
  Relational Operator/1 -> Monostable/1
  Add/1 -> Relational Operator1/1
  Constant/1 -> Relational Operator/2
  Relational Operator2/1 -> Logical Operator/2
  Constant3/1 -> Add/1
  Gain1/1 -> Add1/1, Add/2
  Constant4/1 -> Add1/2
  Logical Operator/1 -> Logical Operator1/1
  Monostable/1 -> Integrator/2
  Relational Operator1/1 -> Logical Operator/1
  Logical Operator1/1 -> Scope2/1, Outport/1
  Vin/1 -> Scope2/2, Scope1/1, Relational Operator/1
  CLK/1 -> Logical Operator1/2
  C/1 -> Integrator/1
  Constant2/1 -> Gain1/1
